simulink library "cooperative"  (Simulink 7.4)
settings: Solver=ode45  SolverMode=SingleTasking  StartTime=0.0  StopTime=10.0  RelTol=1e-3
undefined symbols (not defined in the file): ATRFunctions, g_AssignmentAlgorithm, g_CommandTurnRadius, g_CoordinationDelayDen, g_DefaultWaypointAltitude, g_EntityTypes, g_MaxNumberTargets, g_MaxNumberVehicles, g_MaxReassignmentDeltaTime, g_ObjectMessageIDs, g_OptionSaveDataAVDS, g_SampleTime, g_SensorRollLimitDeg, g_TargetStates, g_Tasks, g_TruthMemory, g_TypeAssignment, g_VehicleInputFiles, g_VehicleMemory, g_VehicleTypes, g_WaypointDefinitions, g_WaypointTypes
libraries: cooperative x23
(part 1 of 3)
settings Model: Creator=RAS  LastModifiedBy=z3311692  ExtModeAutoUpdateStatusClock=off

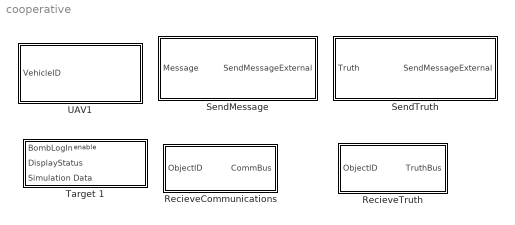
== system cooperative ==
  RecieveCommunications : Subsystem
  RecieveTruth : Subsystem
  SendMessage : Subsystem  mask{ReuseMatrix=growing, MessageTypeStr=ATRSingle}
      mask prompts: ReuseMatrix "Growing or Static memory matrix?"; MessageTypeStr "Select Message Type:"
      mask init:
      | global g_CommunicationMemory;
      | MessageIDIndex = FindMessageIndex(g_CommunicationMemory,MessageTypeStr);
      | MessageType = g_CommunicationMemory.Messages{MessageIDIndex}.ID;
      mask StyleString: popup(growing|static),popup(ETACostToSearch|PositionID|WaypointIndex|TriggerReplan|ATRSingle|ATRTime|TargetStatus|TargetAttacked|ChangedStatus|SendPositionsFlag|TaskBenefits|AuctionData)
  "SendTruth " : Subsystem  mask{ReuseMatrix=static, MessageTypeStr=VehicleState}
      mask prompts: ReuseMatrix "Growing or Static Memory Matrix?"; MessageTypeStr "Select Message Type:"
      mask init:
      | global g_TruthMemory
      | CommunicationsMemory = g_TruthMemory;
      | MessageIDIndex = FindMessageIndex(CommunicationsMemory ,MessageTypeStr);
      | MessageType = CommunicationsMemory.Messages{MessageIDIndex}.ID;
      mask StyleString: popup(growing|static),popup(VehicleState|VehicleIsDead|ChangeVehicleStatus|WeaponsRelease|TargetStatus|TargetState|VehicleStateSaveData|TrackList|ChangeAssignmentFlagSelf)
  Target 1 : Subsystem  AncestorBlock=cooperative/Target 1  TreatAsAtomicUnit=on
  UAV1 : Subsystem  Priority=2

== system cooperative/RecieveCommunications ==
  note: Communications Bus Simulation
      |
      | PURPOSE: Simulate communication subsystem.
      |
      | IMPLEMENTATION:
      | Vehicle-to-vehicle signals are isolated from the CommBus on CommBusSim.  In the case
      | of delayed communications, this is currently implimented with STL deques in the strigger files.
      | Strigger is essentially a trigger taking an arbitrary vector input that can be armed with a scalar
      | delay value...careful with those "enabled" blocks.
      |
      | See m-files:  GetVehicleCommDelay.m and InitializeGlobals.m for the OptionEnableCommDelay.
      |
      | NOTE:  YMMV.
  ObjectID : Inport
  Bus Creator1 : BusCreator  Inputs=24
  S-Function : S-Function  FunctionName=CommunicationsDLL  Parameters='g_CommunicationMemory'  EnableBusSupport=off
  CommBus : Outport
  wires:
  S-Function/24 -> Bus Creator1/24  "AuctionData"
  S-Function/23 -> Bus Creator1/23  "TimeAuctionData"
  S-Function/22 -> Bus Creator1/22  "TaskBenefits"
  S-Function/21 -> Bus Creator1/21  "TimeTaskBenefits"
  S-Function/20 -> Bus Creator1/20  "PositionsFlag"
  S-Function/19 -> Bus Creator1/19  "TimePositionsFlag"
  S-Function/18 -> Bus Creator1/18  "ChangedStatus"
  S-Function/17 -> Bus Creator1/17  "TimeChangedStatus"
  S-Function/16 -> Bus Creator1/16  "TargetAttacked"
  S-Function/15 -> Bus Creator1/15  "TimeTargetAttacked"
  S-Function/14 -> Bus Creator1/14  "TargetStatus"
  S-Function/13 -> Bus Creator1/13  "TimeTargetStatus"
  S-Function/12 -> Bus Creator1/12  "ATRTime"
  S-Function/11 -> Bus Creator1/11  "TimeATRTime"
  S-Function/10 -> Bus Creator1/10  "ATRSingle"
  S-Function/9 -> Bus Creator1/9  "TimeATRSingle"
  S-Function/8 -> Bus Creator1/8  "TriggerReplan"
  S-Function/7 -> Bus Creator1/7  "TimeTriggerReplan"
  S-Function/6 -> Bus Creator1/6  "WaypointIndex"
  S-Function/5 -> Bus Creator1/5  "TimeWaypointIndex"
  S-Function/4 -> Bus Creator1/4  "PositionID"
  S-Function/3 -> Bus Creator1/3  "TimePositionID"
  S-Function/2 -> Bus Creator1/2  "ETACostToSearch"
  S-Function/1 -> Bus Creator1/1  "TimeETACostToSearch"
  ObjectID/1 -> S-Function/1
  Bus Creator1/1 -> CommBus/1  "ExternalComm"

== system cooperative/RecieveTruth ==
  note: Communications Bus Simulation
      |
      | PURPOSE: Simulate communication subsystem.
      |
      | IMPLEMENTATION:
      | Vehicle-to-vehicle signals are isolated from the CommBus on CommBusSim.  In the case
      | of delayed communications, this is currently implimented with STL deques in the strigger files.
      | Strigger is essentially a trigger taking an arbitrary vector input that can be armed with a scalar
      | delay value...careful with those "enabled" blocks.
      |
      | See m-files:  GetVehicleCommDelay.m and InitializeGlobals.m for the OptionEnableCommDelay.
      |
      | NOTE:  YMMV.
  ObjectID : Inport
  Bus Creator1 : BusCreator  Inputs=18
  S-Function : S-Function  FunctionName=CommunicationsDLL  Parameters='g_TruthMemory'  EnableBusSupport=off
  TruthBus : Outport
  wires:
  S-Function/18 -> Bus Creator1/18  "ChangeAssignmentFlagSelf"
  S-Function/17 -> Bus Creator1/17  "TimeChangeAssignmentFlagSelf"
  S-Function/16 -> Bus Creator1/16  "TrackList"
  S-Function/15 -> Bus Creator1/15  "TimeTrackList"
  S-Function/14 -> Bus Creator1/14  "VehicleStateSaveData"
  S-Function/13 -> Bus Creator1/13  "TimeVehicleStateSaveData"
  S-Function/12 -> Bus Creator1/12  "TargetState"
  S-Function/11 -> Bus Creator1/11  "TimeTargetState"
  S-Function/2 -> Bus Creator1/2  "VehicleStates"
  S-Function/1 -> Bus Creator1/1  "TimeVehicleStates"
  S-Function/3 -> Bus Creator1/3  "TimeVehicleIsDead"
  S-Function/4 -> Bus Creator1/4  "VehicleIsDead"
  S-Function/5 -> Bus Creator1/5  "TimeVehicleKilled"
  S-Function/6 -> Bus Creator1/6  "VehicleKilled"
  S-Function/7 -> Bus Creator1/7  "TimeWeaponRelease"
  S-Function/8 -> Bus Creator1/8  "WeaponRelease"
  S-Function/9 -> Bus Creator1/9  "TimeTargetStatus"
  S-Function/10 -> Bus Creator1/10  "TargetStatus"
  ObjectID/1 -> S-Function/1
  Bus Creator1/1 -> TruthBus/1  "ExternalTruth"

== system cooperative/SendMessage ==
  Message : Inport
  Check for Changed Targets : RelationalOperator  Operator=~=  InputSameDT=on
  CreateLastTriggerTime : DataStoreMemory  DataStoreName=LastTriggerTime
  ReadLastTriggerTime : DataStoreRead  DataStoreName=LastTriggerTime  SampleTime=g_SampleTime
  Selector : Selector  IndexOptions=Index vector (dialog)  Indices=2  OutputSizes=1
  SendMessage : Subsystem  TreatAsAtomicUnit=on
  SendMessageExternal : Outport
  wires:
  Message/1 -> Selector/1, SendMessage/2(Message)
  Check for Changed Targets/1 -> SendMessage/Enable
  ReadLastTriggerTime/1 -> Check for Changed Targets/1
  Selector/1 -> Check for Changed Targets/2, SendMessage/1(ReplanTime)
  SendMessage/1(SendMessageExternal) -> SendMessageExternal/1  "SendMessage"

== system cooperative/SendTruth  ==
  Truth : Inport
  Check for Changed Targets : RelationalOperator  Operator=~=  InputSameDT=on
  CreateLastTriggerTime : DataStoreMemory  DataStoreName=LastTriggerTime
  ReadLastTriggerTime : DataStoreRead  DataStoreName=LastTriggerTime  SampleTime=g_SampleTime
  Selector : Selector  IndexOptions=Index vector (dialog)  Indices=2  OutputSizes=1
  SendMessage : Subsystem  TreatAsAtomicUnit=on
  SendMessageExternal : Outport
  wires:
  Selector/1 -> Check for Changed Targets/2, SendMessage/1(ReplanTime)
  ReadLastTriggerTime/1 -> Check for Changed Targets/1
  Check for Changed Targets/1 -> SendMessage/Enable
  Truth/1 -> Selector/1, SendMessage/2(Message)
  SendMessage/1(SendMessageExternal) -> SendMessageExternal/1  "SendMessage"

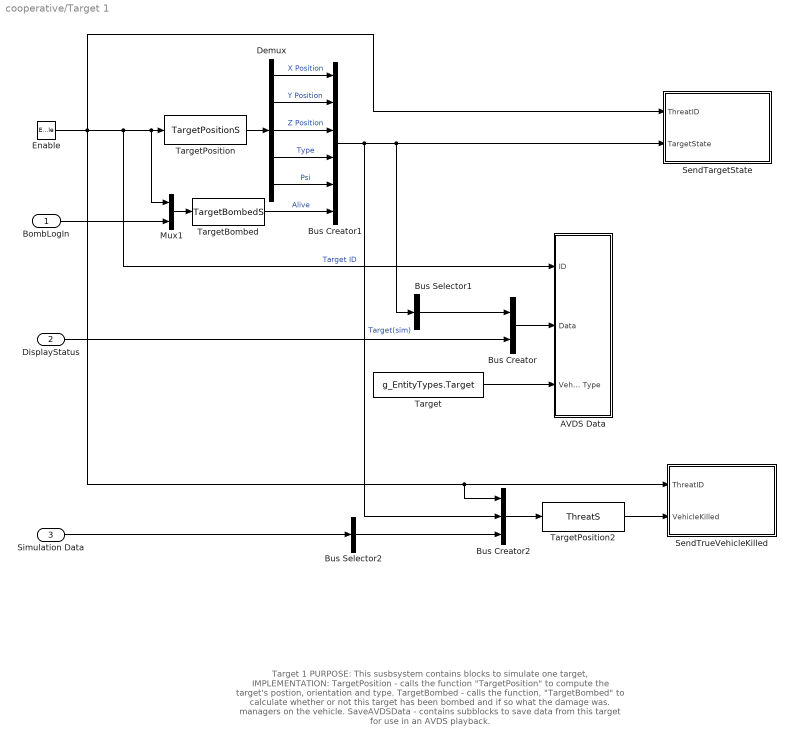
== system cooperative/Target 1 ==
  note: Target 1
      |
      | PURPOSE: This susbsystem contains blocks to simulate one target,
      |
      | IMPLEMENTATION:
      | TargetPosition - calls the function "TargetPosition" to compute the target's postion,
      |      orientation and type.
      | TargetBombed - calls the function, "TargetBombed" to calculate whether or not this
      |      target has been bombed and if so what the damage was.
      |      managers on the vehicle.
      | SaveAVDSData - contains subblocks to save data from this target for use
      |     in an AVDS playback.
  BombLogIn : Inport  SampleTime=g_SampleTime
  DisplayStatus : Inport  Port=2  SampleTime=g_SampleTime
  Simulation Data : Inport  Port=3  SampleTime=g_SampleTime
  Enable : EnablePort  StatesWhenEnabling=reset  ShowOutputPort=on
  AVDS Data : Subsystem
  Bus Creator : BusCreator  Inputs=2
  Bus Creator1 : BusCreator  Inputs=6
  Bus Creator2 : BusCreator  Inputs=3
  Bus Selector1 : BusSelector  OutputSignals=X Position,Y Position,Z Position,Type,Psi  OutputAsBus=on
  Bus Selector2 : BusSelector  OutputSignals=VehicleStates  OutputAsBus=on
  Demux : Demux  Outputs=5
  Mux1 : Mux  Inputs=2
  SendTargetState : Subsystem
  SendTrueVehicleKilled : Subsystem
  Target : Constant  Value=g_EntityTypes.Target
  TargetBombed : S-Function  FunctionName=TargetBombedS  EnableBusSupport=off
  TargetPosition : S-Function  FunctionName=TargetPositionS  EnableBusSupport=off
  TargetPosition2 : S-Function  FunctionName=ThreatS  Parameters=g_MaxNumberVehicles  EnableBusSupport=off
  wires:
  Enable/1 -> AVDS Data/1(ID), Mux1/1, TargetPosition/1, Bus Creator2/1, SendTrueVehicleKilled/1(ThreatID), SendTargetState/1(ThreatID)  "Target ID"
  TargetPosition/1 -> Demux/1
  Target/1 -> AVDS Data/3(Vehicle Type)
  Bus Selector1/1 -> Bus Creator/1
  Demux/1 -> Bus Creator1/1  "X Position"
  Demux/2 -> Bus Creator1/2  "Y Position"
  Demux/3 -> Bus Creator1/3  "Z Position"
  Bus Creator1/1 -> Bus Selector1/1, SendTargetState/2(TargetState), Bus Creator2/2  "Target(sim)"
  Demux/5 -> Bus Creator1/5  "Psi"
  BombLogIn/1 -> Mux1/2
  Demux/4 -> Bus Creator1/4  "Type"
  TargetBombed/1 -> Bus Creator1/6  "Alive"
  Mux1/1 -> TargetBombed/1
  Bus Creator/1 -> AVDS Data/2(Data)
  DisplayStatus/1 -> Bus Creator/2
  TargetPosition2/1 -> SendTrueVehicleKilled/2(VehicleKilled)
  Bus Creator2/1 -> TargetPosition2/1
  Bus Selector2/1 -> Bus Creator2/3
  Simulation Data/1 -> Bus Selector2/1

== system cooperative/UAV1 ==
  note: UAV1
      |
      | PURPOSE: This susbsystem contains blocks to simulate one vehicle,
      |
      | IMPLEMENTATION:
      | Aircraft Dynamics - contains subblocks to implement the vehicle's dynamics
      |      simulation.
      | Embedded Flight Software - contains subblocks to implement the software
      |      managers on the vehicle.
      | SaveAVDSData - contains subblocks to save data from this ehicle for use
      |     in an AVDS playback.
  VehicleID : Inport  SampleTime=g_SampleTime
  Aircraft Dynamics : Subsystem  TreatAsAtomicUnit=on
  Bus Creator : BusCreator  Inputs=1
  Bus Creator1 : BusCreator
  Bus Creator4 : BusCreator  Inputs=1
  Digital Clock : DigitalClock  SampleTime=g_SampleTime
  EmbeddedFlightSoftware : Subsystem
  ReceiveMessages : Subsystem
  ReceiveTruth : Subsystem
  SaveAVDSData : Subsystem
  SendMessages : Subsystem
  SendTruth : Subsystem
  wires:
  ReceiveMessages/1(CommBusSim Out) -> SendMessages/3(CommBus), EmbeddedFlightSoftware/2(ComBusIn)
  Digital Clock/1 -> Bus Creator1/2  "Time"
  EmbeddedFlightSoftware/2(ComBusOut) -> Bus Creator1/4
  EmbeddedFlightSoftware/1(SimBusOut) -> Bus Creator/1
  VehicleID/1 -> ReceiveMessages/1(VehicleID), SaveAVDSData/1(ID), EmbeddedFlightSoftware/5(Enable), ReceiveTruth/1(Vehicle ID), Bus Creator1/1, SendMessages/1(VehicleID), SendTruth/1(VehicleID), Aircraft Dynamics/Enable  "VehicleID"
  Bus Creator/1 -> SaveAVDSData/3(SimBusLocalln), EmbeddedFlightSoftware/3(SimBusLocalIn), SendTruth/3(SimmBusLocal)  "SimBusLocal"
  Bus Creator1/1 -> SaveAVDSData/2(ComBusLocalln), EmbeddedFlightSoftware/4(ComBusLocalIn), Aircraft Dynamics/2(ComBusLocalIn), SendMessages/2(CommBusLocal), SendTruth/2(CommBusLocal)  "ComBusLocal"
  Aircraft Dynamics/1(ComBusOut) -> Bus Creator1/3
  Bus Creator4/1 -> Aircraft Dynamics/1(SimBusIn), EmbeddedFlightSoftware/1(SimBusIn)
  ReceiveTruth/1(TruthBusOut) -> Bus Creator4/1

== system cooperative/SendMessage/SendMessage ==
  ReplanTime : Inport
  Message : Inport  Port=2
  Enable : EnablePort
  Constant : Constant  Value=g_TruthMemory.Transport.MatlabMatrix
  Constant1 : Constant  Value=g_TruthMemory.Transport.TransportType
  Relational Operator : RelationalOperator  Operator===  InputSameDT=on
  SaveLastTriggerTime : DataStoreWrite  DataStoreName=LastTriggerTime  SampleTime=g_SampleTime
  SendMessageMatlab : Subsystem  TreatAsAtomicUnit=on
  SendMessageExternal : Outport
  wires:
  Constant1/1 -> Relational Operator/2
  Constant/1 -> Relational Operator/1
  Relational Operator/1 -> SendMessageMatlab/Enable
  Message/1 -> SendMessageExternal/1, SendMessageMatlab/1(Message)
  ReplanTime/1 -> SaveLastTriggerTime/1

== system cooperative/SendTruth /SendMessage ==
  ReplanTime : Inport
  Message : Inport  Port=2
  Enable : EnablePort
  Constant : Constant  Value=g_TruthMemory.Transport.MatlabMatrix
  Constant1 : Constant  Value=g_TruthMemory.Transport.TransportType
  Relational Operator : RelationalOperator  Operator===  InputSameDT=on
  SaveLastTriggerTime : DataStoreWrite  DataStoreName=LastTriggerTime  SampleTime=g_SampleTime
  SendMessageMatlab : Subsystem  TreatAsAtomicUnit=on
  SendMessageExternal : Outport
  wires:
  ReplanTime/1 -> SaveLastTriggerTime/1
  Message/1 -> SendMessageMatlab/1(Message), SendMessageExternal/1
  Relational Operator/1 -> SendMessageMatlab/Enable
  Constant/1 -> Relational Operator/1
  Constant1/1 -> Relational Operator/2

== system cooperative/Target 1/AVDS Data ==
  note: AVDS Data
      |
      | PURPOSE: Save target state information to a text file that is suitable
      |      for playback in AVDS.
      |
      | IMPLEMENTATION:
      | - Save Target Data for AVDS - calls the function "AVDSData2WorkSpace"
      |      to save the data.
      | - NotAtZero - data saving is enabled when the simulation time is greater
      |      than 0.0 to prevent unitialized data from being written to the file.
      | - EnableDataSaving - reads the global array "OptionSaveDataAVDS" to
      |      enable/disable data saving.
  ID : Inport  SampleTime=g_SampleTime
  Data : Inport  Port=2  SampleTime=g_SampleTime
  Vehicle Type : Inport  Port=3  SampleTime=g_SampleTime
  Digital Clock : DigitalClock  SampleTime=g_SampleTime
  EnableDataSaving : Constant  Value=g_OptionSaveDataAVDS
  Logical Operator : Logic
  NotAtZero : Fcn  Expr=u(1) > 0
  SaveTarget  Data for AVDS : Subsystem  TreatAsAtomicUnit=on
  wires:
  ID/1 -> SaveTarget  Data for AVDS/2(ID)
  Data/1 -> SaveTarget  Data for AVDS/3(Data)
  Digital Clock/1 -> NotAtZero/1, SaveTarget  Data for AVDS/1(Time)
  Vehicle Type/1 -> SaveTarget  Data for AVDS/4(Vehicle Type)
  NotAtZero/1 -> Logical Operator/2
  Logical Operator/1 -> SaveTarget  Data for AVDS/Enable
  EnableDataSaving/1 -> Logical Operator/1

== system cooperative/Target 1/SendTargetState ==
  ThreatID : Inport
  TargetState : Inport  Port=2
  Constant : Constant  Value=0
  CreateTargetState : DataStoreMemory  DataStoreName=TargetState  InitialValue=zeros(6,1)
  Enabled Subsystem : Subsystem  TreatAsAtomicUnit=on
  Logical Operator : Logic  Operator=OR
  Mux2 : Mux  Inputs=3
  ReadTargetState : DataStoreRead  DataStoreName=TargetState  SampleTime=g_SampleTime
  Relational Operator : RelationalOperator  Operator=~=  InputSameDT=on
  Relational Operator1 : RelationalOperator  Operator===  InputSameDT=on
  "SendTruth " : cooperative/SendTruth   ReuseMatrix=static  MessageTypeStr=TargetState
  Terminator : Terminator
  Unit Delay : UnitDelay  SampleTime=g_SampleTime
  wires:
  Relational Operator/1 -> Logical Operator/1
  Enabled Subsystem/1(TimeStamp) -> Unit Delay/1, Mux2/2
  ReadTargetState/1 -> Relational Operator/1
  TargetState/1 -> Enabled Subsystem/1(TargetState), Relational Operator/2, Mux2/3
  ThreatID/1 -> Mux2/1
  Mux2/1 -> "SendTruth "/1
  Logical Operator/1 -> Enabled Subsystem/Enable
  Relational Operator1/1 -> Logical Operator/2
  Constant/1 -> Relational Operator1/1
  Unit Delay/1 -> Relational Operator1/2
  "SendTruth "/1 -> Terminator/1

== system cooperative/Target 1/SendTrueVehicleKilled ==
  ThreatID : Inport
  VehicleKilled : Inport  Port=2
  CreateVehicleKilled : DataStoreMemory  DataStoreName=VehicleKilled  InitialValue=zeros(g_MaxNumberVehicles,1)
  Enabled Subsystem : Subsystem  TreatAsAtomicUnit=on
  Mux2 : Mux
  ReadVehicleKilled : DataStoreRead  DataStoreName=VehicleKilled  SampleTime=g_SampleTime
  Recipients : Constant  Value=g_ObjectMessageIDs.AllVehiclesTypeShifted + 1
  Relational Operator : RelationalOperator  Operator=~=  InputSameDT=on
  "SendTruth " : cooperative/SendTruth   ReuseMatrix=growing  MessageTypeStr=ChangeVehicleStatus
  Terminator : Terminator
  wires:
  Mux2/1 -> "SendTruth "/1
  ThreatID/1 -> Mux2/1
  VehicleKilled/1 -> Mux2/3, Relational Operator/2, Enabled Subsystem/1(VehicleKilled)
  ReadVehicleKilled/1 -> Relational Operator/1
  Enabled Subsystem/1(TimeStamp) -> Mux2/2
  Relational Operator/1 -> Enabled Subsystem/Enable
  Recipients/1 -> Mux2/4
  "SendTruth "/1 -> Terminator/1

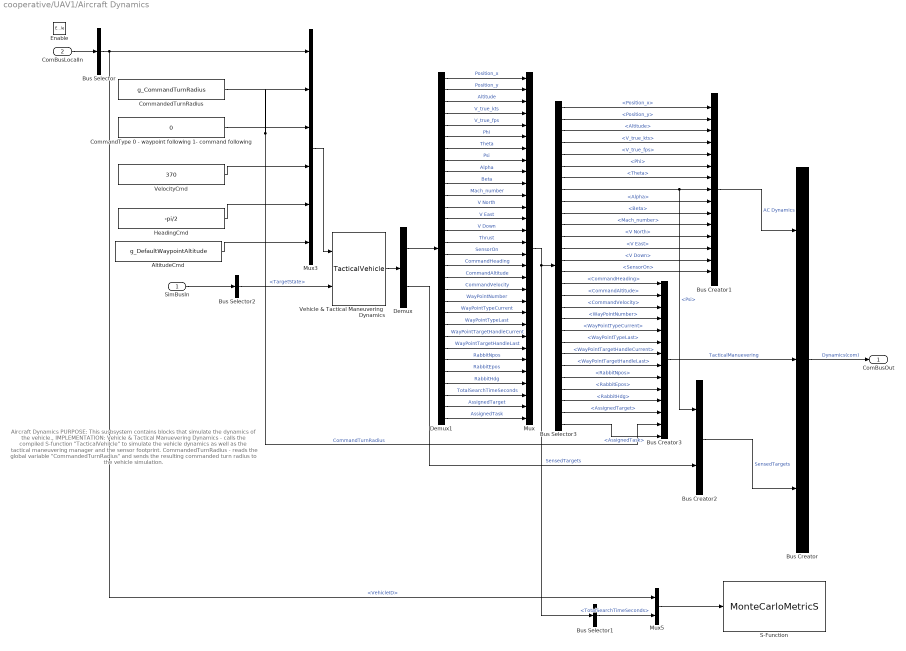
== system cooperative/UAV1/Aircraft Dynamics ==
  note: Aircraft Dynamics
      |
      | PURPOSE: This susbsystem contains blocks that simulate the dynamics of the vehicle.,
      |
      | IMPLEMENTATION:
      | Vehicle & Tactical Manuevering Dynamics - calls the compiled S-function "TacticalVehilcle"
      |      to simulate the vehicle dynamics as well as the tactical maneuvering manager and the
      |      sensor footprint.
      | CommandedTurnRadius - reads the global variable "CommandedTurnRadius" and sends
      |      the resulting commanded turn radius to the vehicle simulation.
  SimBusIn : Inport  SampleTime=g_SampleTime
  ComBusLocalIn : Inport  Port=2  SampleTime=g_SampleTime
  Enable : EnablePort
  AltitudeCmd : Constant  Value=g_DefaultWaypointAltitude
  Bus Creator : BusCreator  Inputs=3
  Bus Creator1 : BusCreator  Inputs=15
  Bus Creator2 : BusCreator  Inputs=2
  Bus Creator3 : BusCreator  Inputs=14
  Bus Selector : BusSelector  OutputSignals=VehicleID
  Bus Selector1 : BusSelector  OutputSignals=TotalSearchTimeSeconds
  Bus Selector2 : BusSelector  OutputSignals=ExternalTruth.TargetState
  Bus Selector3 : BusSelector  OutputSignals=Position_x,Position_y,Altitude,V_true_kts,V_true_fps,Phi,Theta,Psi,Alpha,Beta,Mach_number,V North,V East,V Down,SensorOn,CommandHeading,CommandAltitude,CommandVelocity,WayPointNumber,WayPointTypeCurrent,WayPointTypeLast,WayPointTargetHandleCurrent,WayPointTargetHandleLast,RabbitNpos,RabbitEpos,RabbitHdg,AssignedTarget,AssignedTask
  CommandType 0 - waypoint following 1- command following : Constant  Value=0
  CommandedTurnRadius : Constant  Value=g_CommandTurnRadius
  Demux : Demux  Outputs=[30 g_MaxNumberTargets]
  Demux1 : Demux  Outputs=30
  HeadingCmd : Constant  Value=-pi/2
  Mux : Mux  Inputs=30
  Mux3 : Mux  Inputs=6
  Mux5 : Mux  Inputs=2
  S-Function : S-Function  FunctionName=MonteCarloMetricS  Parameters='TotalSearchTimeSeconds'  EnableBusSupport=off
  Vehicle & Tactical Maneuvering  Dynamics : S-Function  FunctionName=TacticalVehicle  Parameters=0,g_MaxNumberTargets,g_SensorRollLimitDeg,g_WaypointDefinitions.NumberEntries,g_VehicleInputFiles  EnableBusSupport=off
  VelocityCmd : Constant  Value=370
  ComBusOut : Outport
  wires:
  Bus Selector1/1 -> Mux5/2  "<TotalSearchTimeSeconds>"
  Mux5/1 -> S-Function/1
  Demux1/25 -> Mux/25  "RabbitNpos"
  Demux1/30 -> Mux/30  "AssignedTask"
  ComBusLocalIn/1 -> Bus Selector/1
  SimBusIn/1 -> Bus Selector2/1
  Bus Creator3/1 -> Bus Creator/2  "TacticalManuevering"
  Mux/1 -> Bus Selector1/1, Bus Selector3/1
  Bus Selector3/15 -> Bus Creator1/15  "<SensorOn>"
  Bus Creator1/1 -> Bus Creator/1  "AC Dynamics"
  Bus Selector3/14 -> Bus Creator1/14  "<V Down>"
  Bus Selector3/13 -> Bus Creator1/13  "<V East>"
  Bus Selector3/12 -> Bus Creator1/12  "<V North>"
  Bus Selector3/11 -> Bus Creator1/11  "<Mach_number>"
  Bus Selector3/10 -> Bus Creator1/10  "<Beta>"
  Bus Selector3/9 -> Bus Creator1/9  "<Alpha>"
  Bus Selector3/8 -> Bus Creator1/8, Bus Creator2/1  "<Psi>"
  Bus Selector3/7 -> Bus Creator1/7  "<Theta>"
  Bus Selector3/6 -> Bus Creator1/6  "<Phi>"
  Bus Selector3/5 -> Bus Creator1/5  "<V_true_fps>"
  Bus Selector3/4 -> Bus Creator1/4  "<V_true_kts>"
  Bus Selector3/3 -> Bus Creator1/3  "<Altitude>"
  Bus Selector3/2 -> Bus Creator1/2  "<Position_y>"
  Bus Selector3/1 -> Bus Creator1/1  "<Position_x>"
  Demux1/29 -> Mux/29  "AssignedTarget"
  Demux1/27 -> Mux/27  "RabbitHdg"
  Demux1/26 -> Mux/26  "RabbitEpos"
  Demux1/22 -> Mux/22  "WayPointTypeLast"
  Demux1/21 -> Mux/21  "WayPointTypeCurrent"
  Demux1/20 -> Mux/20  "WayPointNumber"
  Demux1/19 -> Mux/19  "CommandVelocity"
  Demux1/18 -> Mux/18  "CommandAltitude"
  Demux1/17 -> Mux/17  "CommandHeading"
  Demux1/16 -> Mux/16  "SensorOn"
  Demux1/15 -> Mux/15  "Thrust"
  Demux1/14 -> Mux/14  "V Down"
  Demux1/13 -> Mux/13  "V East"
  Demux1/12 -> Mux/12  "V North"
  Demux1/11 -> Mux/11  "Mach_number"
  Demux1/10 -> Mux/10  "Beta"
  Demux1/9 -> Mux/9  "Alpha"
  Demux1/8 -> Mux/8  "Psi"
  Demux1/7 -> Mux/7  "Theta"
  Demux1/6 -> Mux/6  "Phi"
  Demux1/5 -> Mux/5  "V_true_fps"
  Demux1/4 -> Mux/4  "V_true_kts"
  Demux1/2 -> Mux/2  "Position_y"
  Demux1/1 -> Mux/1  "Position_x"
  Demux1/3 -> Mux/3  "Altitude"
  Demux/2 -> Bus Creator2/2  "SensedTargets"
  Demux/1 -> Demux1/1
  Bus Creator2/1 -> Bus Creator/3  "SensedTargets"
  Bus Creator/1 -> ComBusOut/1  "Dynamics(com)"
  CommandedTurnRadius/1 -> Bus Creator3/13, Mux3/2  "CommandTurnRadius"
  Bus Selector/1 -> Mux5/1, Mux3/1  "<VehicleID>"
  Vehicle & Tactical Maneuvering  Dynamics/1 -> Demux/1
  Bus Selector2/1 -> Vehicle & Tactical Maneuvering  Dynamics/2  "<TargetState>"
  Mux3/1 -> Vehicle & Tactical Maneuvering  Dynamics/1
  Demux1/23 -> Mux/23  "WayPointTargetHandleCurrent"
  Demux1/24 -> Mux/24  "WayPointTargetHandleLast"
  Demux1/28 -> Mux/28  "TotalSearchTimeSeconds"
  Bus Selector3/16 -> Bus Creator3/1  "<CommandHeading>"
  Bus Selector3/17 -> Bus Creator3/2  "<CommandAltitude>"
  Bus Selector3/18 -> Bus Creator3/3  "<CommandVelocity>"
  Bus Selector3/19 -> Bus Creator3/4  "<WayPointNumber>"
  Bus Selector3/20 -> Bus Creator3/5  "<WayPointTypeCurrent>"
  Bus Selector3/21 -> Bus Creator3/6  "<WayPointTypeLast>"
  Bus Selector3/22 -> Bus Creator3/7  "<WayPointTargetHandleCurrent>"
  Bus Selector3/23 -> Bus Creator3/8  "<WayPointTargetHandleLast>"
  Bus Selector3/24 -> Bus Creator3/9  "<RabbitNpos>"
  Bus Selector3/25 -> Bus Creator3/10  "<RabbitEpos>"
  Bus Selector3/26 -> Bus Creator3/11  "<RabbitHdg>"
  Bus Selector3/27 -> Bus Creator3/12  "<AssignedTarget>"
  Bus Selector3/28 -> Bus Creator3/14  "<AssignedTask>"
  CommandType 0 - waypoint following 1- command following/1 -> Mux3/3
  VelocityCmd/1 -> Mux3/4
  HeadingCmd/1 -> Mux3/5
  AltitudeCmd/1 -> Mux3/6

== system cooperative/UAV1/EmbeddedFlightSoftware ==
  note: EmbeddedFlightSoftware
      |
      | PURPOSE: This susbsystem contains subsystems to implement the software
      |      managers on the vehicle,
      |
      | IMPLEMENTATION:
      | - Sensor Manager -  This manager is used to perform all of the functions
      |      necessary to monitor the sensors and process sensed data.
      | - TargetManager - Tracks and updates the status of all kown targets.
      | - WeaponsManager - Selects a weapon and then simulates its deployment.
      | - CooperationManager - This manager is used to facilitate cooperation
      |      between the vehicles. At this time the only function implemented is the
      |      Assginment manager.
      | - RouteManager - This manager is used to plan and select the route
      |      for the vehicle to fly. Part of the functionality is calculation of the lowest
      |      cost route to all known targets, based on each target's state.
  SimBusIn : Inport  SampleTime=g_SampleTime
  ComBusIn : Inport  Port=2  SampleTime=g_SampleTime
  SimBusLocalIn : Inport  Port=3  SampleTime=g_SampleTime
  ComBusLocalIn : Inport  Port=4  SampleTime=g_SampleTime
  Enable : Inport  Port=5  SampleTime=g_SampleTime
  Bus Creator : BusCreator  Inputs=3
  Bus Creator1 : BusCreator  Inputs=5
  CooperationManager : Subsystem
  RouteManager : Subsystem
  SensorManager : Subsystem
  TargetManager : Subsystem
  TimeLastReplan1 : DataStoreMemory  DataStoreName=TimeLastReplan
  WeaponsManager : Subsystem  TreatAsAtomicUnit=on
  SimBusOut : Outport
  ComBusOut : Outport  Port=2
  wires:
  Enable/1 -> RouteManager/5(Enable), CooperationManager/4(Enable), WeaponsManager/Enable, SensorManager/4(Enable), TargetManager/4(Enable)
  RouteManager/2(ComBusOut) -> Bus Creator1/5
  CooperationManager/1(ComBusOut) -> Bus Creator1/4
  WeaponsManager/2(ComBusOut) -> Bus Creator1/3
  TargetManager/1(ComBusOut) -> Bus Creator1/2
  SensorManager/1(ComBusOut) -> Bus Creator1/1
  RouteManager/1(SimBusOut) -> Bus Creator/3
  WeaponsManager/1(SimBusOut) -> Bus Creator/1
  Bus Creator/1 -> SimBusOut/1  "EFS(sim)"
  Bus Creator1/1 -> ComBusOut/1  "EFS(com)"
  SimBusIn/1 -> TargetManager/1(SimBusIn), SensorManager/1(SimBusIn), CooperationManager/1(SimBusIn), RouteManager/1(SimBusIn)
  ComBusIn/1 -> TargetManager/2(ComBusIn), SensorManager/2(ComBusIn), CooperationManager/2(ComBusIn), RouteManager/2(ComBusIn)
  SimBusLocalIn/1 -> RouteManager/3(SimBusLocalIn)
  ComBusLocalIn/1 -> WeaponsManager/1(ComBusLocalIn), TargetManager/3(ComBusLocalIn), SensorManager/3(ComBusLocalIn), CooperationManager/3(ComBusLocalIn), RouteManager/4(ComBusLocalIn)
  CooperationManager/2(SimBusOut) -> Bus Creator/2

== system cooperative/UAV1/ReceiveMessages ==
  VehicleID : Inport
  RecieveCommunications : cooperative/RecieveCommunications
      settings: RTWFcnNameOpts=Auto  RTWFileNameOpts=Auto
  Sum : Sum  Inputs=|++  SaturateOnIntegerOverflow=on  InputSameDT=on  OutDataTypeStr=Inherit: Same as first input
  VehicleOffset : Constant  Value=g_ObjectMessageIDs.VehicleIDOffset
  CommBusSim Out : Outport
  wires:
  RecieveCommunications/1 -> CommBusSim Out/1
  VehicleID/1 -> Sum/1
  VehicleOffset/1 -> Sum/2
  Sum/1 -> RecieveCommunications/1

== system cooperative/UAV1/ReceiveTruth ==
  Vehicle ID : Inport
  ImplementNewAssignment : Subsystem
  RecieveTruth : cooperative/RecieveTruth
      settings: RTWFcnNameOpts=Auto  RTWFileNameOpts=Auto
  Sum : Sum  Inputs=|+|+|  SaturateOnIntegerOverflow=on  InputSameDT=on  OutDataTypeStr=Inherit: Same as first input
  VehicleOffset : Constant  Value=g_ObjectMessageIDs.VehicleIDOffset
  TruthBusOut : Outport
  wires:
  RecieveTruth/1 -> TruthBusOut/1, ImplementNewAssignment/2(TruthBus)
  Vehicle ID/1 -> ImplementNewAssignment/1(VehicleID), Sum/2
  Sum/1 -> RecieveTruth/1
  VehicleOffset/1 -> Sum/1

== system cooperative/UAV1/SaveAVDSData ==
  note: AVDS Data
      |
      | PURPOSE: Save vehicle state information to a
      | text file that is suitable for playback in AVDS.
      |
      | IMPLEMENTATION:
      | - SaveVehicleData for AVDS - calls the function "AVDSData2WorkSpace"
      |      to save the data.
      | - NotAtZero - data saving is enabled when the simulation time is greater
      |      than 0.0 to prevent unitialized data from being written to the file.
      | -EnableDataSaving - reads the global array "OptionSaveDataAVDS" to
      |      enables/disables saving data forAVDS.
  ID : Inport  SampleTime=g_SampleTime
  ComBusLocalln : Inport  Port=2  SampleTime=g_SampleTime
  SimBusLocalln : Inport  Port=3  SampleTime=g_SampleTime
  Aircraft : Constant  Value=g_EntityTypes.Aircraft
  Bus Selector2 : BusSelector  OutputSignals=Dynamics(com).AC Dynamics.Position_x,Dynamics(com).AC Dynamics.Position_y,Dynamics(com).AC Dynamics.Altitude,Dynamics(com).AC Dynamics.Phi,Dynamics(com).AC Dynamics.Theta,Dynamics(com).AC Dynamics.Psi,Dynamics(com).AC Dynamics.Alpha,Dynamics(com).AC Dynamics.Beta,Dynamics(com).AC Dynamics.V_true_fps,Dynamics(com).AC Dynamics.Mach_number,Dynamics(com).TacticalManuevering.AssignedTarget,Dynamics(com).TacticalManuevering.AssignedTask,Dynamics(com).TacticalManuevering.RabbitNpos,Dynamics(com).TacticalManuevering.RabbitEpos,Dynamics(com).TacticalManuevering.RabbitHdg,Dynamics(com).TacticalManuevering.CommandAltitude,Dynamics(com).AC Dynamics.SensorOn  OutputAsBus=on
  Bus Selector3 : BusSelector  OutputSignals=EFS(sim).RouteManager(sim).VehicleFinished.Vehicle FinishedNoDelay
  Digital Clock : DigitalClock  SampleTime=g_SampleTime
  "EnableDataSaving " : Constant  Value=g_OptionSaveDataAVDS
  Logical Operator : Logic  Inputs=3
  Mux4 : Mux  Inputs=2
  NotAtZero : Fcn  Expr=u(1) > g_SampleTime
  SaveVehicleData for AVDS : Subsystem  TreatAsAtomicUnit=on
  wires:
  NotAtZero/1 -> Logical Operator/3
  Aircraft/1 -> SaveVehicleData for AVDS/4(Vehicle Type)
  Digital Clock/1 -> SaveVehicleData for AVDS/1(Time), NotAtZero/1
  SimBusLocalln/1 -> Bus Selector3/1
  ComBusLocalln/1 -> Bus Selector2/1
  ID/1 -> SaveVehicleData for AVDS/2(ID), Logical Operator/2
  Logical Operator/1 -> SaveVehicleData for AVDS/Enable
  "EnableDataSaving "/1 -> Logical Operator/1
  Bus Selector2/1 -> Mux4/1
  Bus Selector3/1 -> Mux4/2  "<Vehicle FinishedNoDelay>"
  Mux4/1 -> SaveVehicleData for AVDS/3(Data)

== system cooperative/UAV1/SendMessages ==
  note: Messages must have elements starting with vehicleid,timestamp,...
  VehicleID : Inport
  CommBusLocal : Inport  Port=2
  CommBus : Inport  Port=3
  SendATRSingle : Subsystem
  SendATRTime : Subsystem
  SendAuctionData : Subsystem
  SendChangedStatus : Subsystem
  SendETAsCostsReturnToSearch : Subsystem
  SendPositionFlag : Subsystem
  SendPositionID : Subsystem
  SendTargetAttacked : Subsystem
  SendTargetStatus : Subsystem
  SendTaskBenefits : Subsystem
  SendTriggerReplan : Subsystem  Priority=1
  SendWaypointNumber : Subsystem
  wires:
  CommBus/1 -> SendPositionFlag/3(CommBus), SendPositionID/3(CommBus)
  CommBusLocal/1 -> SendATRTime/2(CommBusLocal), SendATRSingle/2(CommBusLocal), SendETAsCostsReturnToSearch/2(CommBusLocal), SendTriggerReplan/2(CommBusLocal), SendAuctionData/2(CommBusLocal), SendTaskBenefits/2(CommBusLocal), SendPositionFlag/2(CommBusLocal), SendPositionID/2(CommBusLocal), SendTargetStatus/2(CommBusLocal), SendTargetAttacked/2(CommBusLocal), SendChangedStatus/2(CommBusLocal), SendWaypointNumber/2(CommBusLocal)
  VehicleID/1 -> SendETAsCostsReturnToSearch/1(VehicleID), SendTriggerReplan/1(VehicleID), SendATRTime/1(VehicleID), SendAuctionData/1(VehicleID), SendTaskBenefits/1(VehicleID), SendPositionFlag/1(VehicleID), SendPositionID/1(VehicleID), SendTargetStatus/1(VehicleID), SendTargetAttacked/1(VehicleID), SendChangedStatus/1(VehicleID), SendWaypointNumber/1(VehicleID), SendATRSingle/1(VehicleID)

== system cooperative/UAV1/SendTruth ==
  note: Messages must have elements starting with vehicleid,timestamp,...
  VehicleID : Inport
  CommBusLocal : Inport  Port=2
  SimmBusLocal : Inport  Port=3
  SendNewAssignment : Subsystem
  SendTargetStatus : Subsystem
  SendTrackList : Subsystem
  SendTrueVehicleState : Subsystem
  SendVehicleIsDead : Subsystem
  SendWeaponsRelease : Subsystem
  VehicleStateSaveData : Subsystem
  wires:
  VehicleID/1 -> SendVehicleIsDead/1(VehicleID), SendWeaponsRelease/1(VehicleID), SendTargetStatus/1(VehicleID), VehicleStateSaveData/1(VehicleID), SendTrackList/1(VehicleID), SendTrueVehicleState/1(VehicleID), SendNewAssignment/1(VehicleID)
  CommBusLocal/1 -> SendTrueVehicleState/2(CommBusLocal), SendTargetStatus/2(CommBusLocal), VehicleStateSaveData/2(CommBusLocal), SendTrackList/2(CommBusLocal)
  SimmBusLocal/1 -> SendWeaponsRelease/2(SimmBusLocal), SendVehicleIsDead/2(SimmBusLocal), VehicleStateSaveData/3(SimmBusLocal), SendTrueVehicleState/3(SimmBusLocal), SendNewAssignment/2(SimmBusLocal)

== system cooperative/SendMessage/SendMessage/SendMessageMatlab ==
  Message : Inport
  Enable : EnablePort
  SendMessageS : S-Function  FunctionName=SendMessageS  Parameters='g_CommunicationMemory',MessageType,ReuseMatrix  EnableBusSupport=off
  wires:
  Message/1 -> SendMessageS/1

== system cooperative/SendTruth /SendMessage/SendMessageMatlab ==
  Message : Inport
  Enable : EnablePort
  SendMessageS : S-Function  FunctionName=SendMessageS  Parameters='g_TruthMemory',MessageType,ReuseMatrix  EnableBusSupport=off
  wires:
  Message/1 -> SendMessageS/1

== system cooperative/Target 1/AVDS Data/SaveTarget  Data for AVDS ==
  note: SaveTargetData for AVDS
      |
      | PURPOSE: Saves target state information to a text file that is suitable
      |      for playback in AVDS.
      | IMPLEMENTATION:
      | - AVDSData2WorkSpace - calls the M-function "AVDSData2WorkSpace"
      |      to save the data.
  Time : Inport  SampleTime=g_SampleTime
  ID : Inport  Port=2  SampleTime=g_SampleTime
  Data : Inport  Port=3  SampleTime=g_SampleTime
  Vehicle Type : Inport  Port=4  SampleTime=g_SampleTime
  Enable : EnablePort
  AVDSData2WorkSpaceS : S-Function  FunctionName=AVDSData2WorkSpaceS  EnableBusSupport=off
  Mux1 : Mux
  wires:
  Mux1/1 -> AVDSData2WorkSpaceS/1
  Time/1 -> Mux1/2
  ID/1 -> Mux1/1
  Data/1 -> Mux1/3
  Vehicle Type/1 -> Mux1/4

== system cooperative/Target 1/SendTargetState/Enabled Subsystem ==
  TargetState : Inport
  Enable : EnablePort
  Digital Clock : DigitalClock  SampleTime=g_SampleTime
  SaveTargetState : DataStoreWrite  DataStoreName=TargetState  SampleTime=g_SampleTime
  TimeStamp : Outport
  wires:
  Digital Clock/1 -> TimeStamp/1
  TargetState/1 -> SaveTargetState/1

== system cooperative/Target 1/SendTrueVehicleKilled/Enabled Subsystem ==
  VehicleKilled : Inport
  Enable : EnablePort
  Digital Clock : DigitalClock  SampleTime=g_SampleTime
  SaveVehicleKilled : DataStoreWrite  DataStoreName=VehicleKilled  SampleTime=g_SampleTime
  TimeStamp : Outport
  wires:
  VehicleKilled/1 -> SaveVehicleKilled/1
  Digital Clock/1 -> TimeStamp/1

== system cooperative/UAV1/EmbeddedFlightSoftware/CooperationManager ==
  note: Cooperation Manager
      |
      | PURPOSE: This manager is used to facilitate cooperation
      |      between the vehicles. At this time the only function
      |      implemented is the Assginment manager which calculates
      |      vehicle /task assignments.
      |
      | IMPLEMENTATION:
      | - Coordination Timing - adds a time delay before the assignment
      |      calculation to give other vehicles time to generate new plans.
      | - Calculate Assignment - this subsystem contains blocks used to
      |      calculate the vehicle/task assignments. This block is enabled
      |      by the signal "New Plans", after the Coordination Timing delay.
  SimBusIn : Inport  SampleTime=g_SampleTime
  ComBusIn : Inport  Port=2  SampleTime=g_SampleTime
  ComBusLocalIn : Inport  Port=3  SampleTime=g_SampleTime
  Enable : Inport  Port=4  SampleTime=g_SampleTime
  Bus Creator : BusCreator  Inputs=3
  Bus Creator1 : BusCreator  Inputs=1
  Calculate Assignment : Subsystem  TreatAsAtomicUnit=on
  Enable Reassignment : Subsystem
  Task List : Subsystem
  Terminator : Terminator
  ComBusOut : Outport
  SimBusOut : Outport  Port=2
  wires:
  Calculate Assignment/3(AuctionData) -> Bus Creator/3
  Calculate Assignment/2(Algorithm Data) -> Bus Creator/2
  Task List/1(UnassignTaskFlag) -> Terminator/1
  SimBusIn/1 -> Calculate Assignment/3(SimBusIn)
  Enable Reassignment/1(Enable Reassignment) -> Calculate Assignment/Enable
  Enable/1 -> Enable Reassignment/1(Enable)
  ComBusLocalIn/1 -> Task List/1(ComBusLocalIn), Enable Reassignment/2(ComBusLocalIn), Calculate Assignment/1(ComBusLocalIn)  "Local Bus"
  ComBusIn/1 -> Enable Reassignment/3(ComBusIn), Calculate Assignment/2(ComBusIn)
  Calculate Assignment/1(Local Assignment) -> Bus Creator/1  "Assignment"
  Bus Creator/1 -> ComBusOut/1  "CooperationManager(com)"
  Calculate Assignment/4(NewAssignmetTime) -> Bus Creator1/1  "NewAssignmentTime"
  Bus Creator1/1 -> SimBusOut/1  "CooperationManager(com)"

== system cooperative/UAV1/EmbeddedFlightSoftware/RouteManager ==
  note: Route Manager
      |
      | PURPOSE: This manager is used to plan and select the route for the
      |      vehicle to fly.
      |
      | Implementation:
      | - Replan - when enabled, calculates the lowest cost route to all known targets,
      |      based on each target's state. Replan is enabled If any of the vehicles report
      |      "Task Finished" or if any of the targets change state,
      | - RouteSelection - calls the function "RouteSelection" to implement waypoints
      |      for the route selected for this vehicle during the vehicle/target assignment in
      |      the cooperation manager.
      | - Task Status - monitors the status of the vehicle's assigned task.
  SimBusIn : Inport  SampleTime=g_SampleTime
  ComBusIn : Inport  Port=2  SampleTime=g_SampleTime
  SimBusLocalIn : Inport  Port=3  SampleTime=g_SampleTime
  ComBusLocalIn : Inport  Port=4  SampleTime=g_SampleTime
  Enable : Inport  Port=5  SampleTime=g_SampleTime
  Bus Creator : BusCreator  Inputs=1
  Bus Creator1 : BusCreator  Inputs=3
  Constant : Constant  Value=g_AssignmentAlgorithm
  Constant1 : Constant  Value=g_TypeAssignment.CapTransShip
  Logical Operator : Logic
  Relational Operator : RelationalOperator  Operator===  InputSameDT=on
  ReplanSingle : Subsystem
  Task Status : Subsystem
  SimBusOut : Outport
  ComBusOut : Outport  Port=2
  wires:
  Constant1/1 -> Relational Operator/2
  Constant/1 -> Relational Operator/1
  Relational Operator/1 -> Logical Operator/1
  Logical Operator/1 -> ReplanSingle/3(Enable)
  Enable/1 -> Task Status/2(Enable), Logical Operator/2
  ReplanSingle/1(NewPlans) -> Bus Creator1/1
  Bus Creator/1 -> SimBusOut/1  "RouteManager(sim)"
  ComBusIn/1 -> ReplanSingle/1(ComBusIn)
  Task Status/1(Task Status) -> Bus Creator1/3
  Task Status/2(Vehicle Finished) -> Bus Creator/1
  SimBusIn/1 -> ReplanSingle/4(SimBusIn), Task Status/3(SimBusIn)
  ReplanSingle/2(ReplanETAsCosts) -> Bus Creator1/2
  Bus Creator1/1 -> ComBusOut/1  "RouteManager(com)"
  ComBusLocalIn/1 -> Task Status/1(Local (Comm)), ReplanSingle/2(ComBusLocalIn)  "Local Bus"
  SimBusLocalIn/1 -> ReplanSingle/5(SimBusLocalIn)  "Vehicle (Sim)"

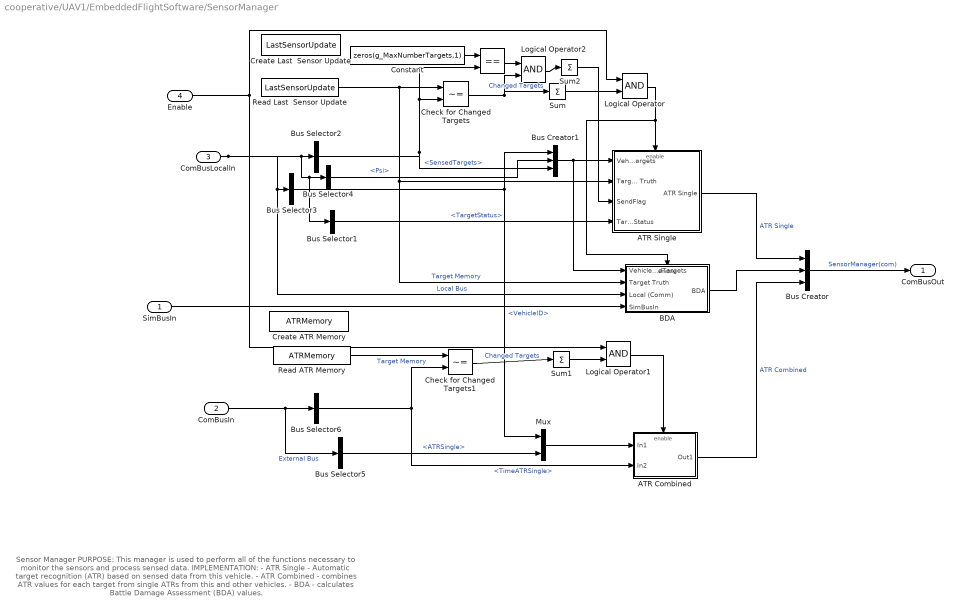
== system cooperative/UAV1/EmbeddedFlightSoftware/SensorManager ==
  note: Sensor Manager
      |
      | PURPOSE: This manager is used to perform all of the functions
      | necessary to monitor the sensors and process sensed data.
      |
      | IMPLEMENTATION:
      | - ATR Single - Automatic target recognition (ATR) based on sensed data
      |      from this vehicle.
      | - ATR Combined - combines ATR values for each target from single ATRs
      |      from this and other vehicles.
      | - BDA - calculates Battle Damage Assessment (BDA) values.
  SimBusIn : Inport  SampleTime=g_SampleTime
  ComBusIn : Inport  Port=2  SampleTime=g_SampleTime
  ComBusLocalIn : Inport  Port=3  SampleTime=g_SampleTime
  Enable : Inport  Port=4  SampleTime=g_SampleTime
  " " : RelationalOperator  Operator===  InputSameDT=on
  ATR Combined : Subsystem  TreatAsAtomicUnit=on
  ATR Single : Subsystem  TreatAsAtomicUnit=on
  BDA : Subsystem  TreatAsAtomicUnit=on
  Bus Creator : BusCreator  Inputs=3
  Bus Creator1 : BusCreator  Inputs=3
  Bus Selector1 : BusSelector  OutputSignals=EFS(com).TargetManager(com).Target Status.TargetStatus
  Bus Selector2 : BusSelector  OutputSignals=Dynamics(com).SensedTargets.SensedTargets
  Bus Selector3 : BusSelector  OutputSignals=VehicleID
  Bus Selector4 : BusSelector  OutputSignals=Dynamics(com).AC Dynamics.Psi
  Bus Selector5 : BusSelector  OutputSignals=ATRSingle
  Bus Selector6 : BusSelector  OutputSignals=TimeATRSingle
  Check for Changed Targets : RelationalOperator  Operator=~=  InputSameDT=on
  Check for Changed Targets1 : RelationalOperator  Operator=~=  InputSameDT=on
  Constant : Constant  Value=zeros(g_MaxNumberTargets,1)
  Create ATR Memory : DataStoreMemory  DataStoreName=ATRMemory  InitialValue=1
  Create Last  Sensor Update : DataStoreMemory  DataStoreName=LastSensorUpdate  InitialValue=zeros(g_MaxNumberTargets,1)
  Logical Operator : Logic
  Logical Operator1 : Logic
  Logical Operator2 : Logic
  Mux : Mux  Inputs=2
  Read ATR Memory : DataStoreRead  DataStoreName=ATRMemory  SampleTime=g_SampleTime
  Read Last  Sensor Update : DataStoreRead  DataStoreName=LastSensorUpdate  SampleTime=g_SampleTime
  Sum : Sum  Inputs=|+  SaturateOnIntegerOverflow=on  InputSameDT=on  OutDataTypeStr=Inherit: Same as first input
  Sum1 : Sum  Inputs=|+  SaturateOnIntegerOverflow=on  InputSameDT=on  OutDataTypeStr=Inherit: Same as first input
  Sum2 : Sum  Inputs=|+  SaturateOnIntegerOverflow=on  InputSameDT=on  OutDataTypeStr=Inherit: Same as first input
  ComBusOut : Outport
  wires:
  Bus Selector1/1 -> ATR Single/4(TargetStatus)  "<TargetStatus>"
  Sum2/1 -> ATR Single/3(SendFlag)
  Logical Operator2/1 -> Sum2/1
  " "/1 -> Logical Operator2/1
  Constant/1 -> " "/1
  Enable/1 -> Logical Operator1/1, Logical Operator/1
  Logical Operator1/1 -> ATR Combined/Enable
  Sum1/1 -> Logical Operator1/2
  Logical Operator/1 -> BDA/Enable, ATR Single/Enable
  Sum/1 -> Logical Operator/2
  ATR Single/1(ATR Single) -> Bus Creator/1  "ATR Single"
  BDA/1(BDA) -> Bus Creator/2
  Bus Creator/1 -> ComBusOut/1  "SensorManager(com)"
  ATR Combined/1(Out1) -> Bus Creator/3  "ATR Combined"
  Bus Selector6/1 -> ATR Combined/2(In2), Check for Changed Targets1/2  "<TimeATRSingle>"
  Mux/1 -> ATR Combined/1(In1)
  Bus Selector5/1 -> Mux/2  "<ATRSingle>"
  ComBusIn/1 -> Bus Selector5/1, Bus Selector6/1  "External Bus"
  Bus Selector4/1 -> Bus Creator1/2  "<Psi>"
  Bus Selector3/1 -> Mux/1, Bus Creator1/1  "<VehicleID>"
  Bus Selector2/1 -> " "/2, Check for Changed Targets/2, Bus Creator1/3  "<SensedTargets>"
  Bus Creator1/1 -> BDA/1(VehicleID Psi SensedTargets), ATR Single/1(VehicleID Psi SensedTargets)
  ComBusLocalIn/1 -> BDA/3(Local (Comm)), Bus Selector3/1, Bus Selector1/1, Bus Selector4/1, Bus Selector2/1  "Local Bus"
  Read ATR Memory/1 -> Check for Changed Targets1/1  "Target Memory"
  Check for Changed Targets1/1 -> Sum1/1  "Changed Targets"
  Read Last  Sensor Update/1 -> BDA/2(Target Truth), ATR Single/2(Target Truth), Check for Changed Targets/1  "Target Memory"
  Check for Changed Targets/1 -> Logical Operator2/2, Sum/1  "Changed Targets"
  SimBusIn/1 -> BDA/4(SimBusIn)

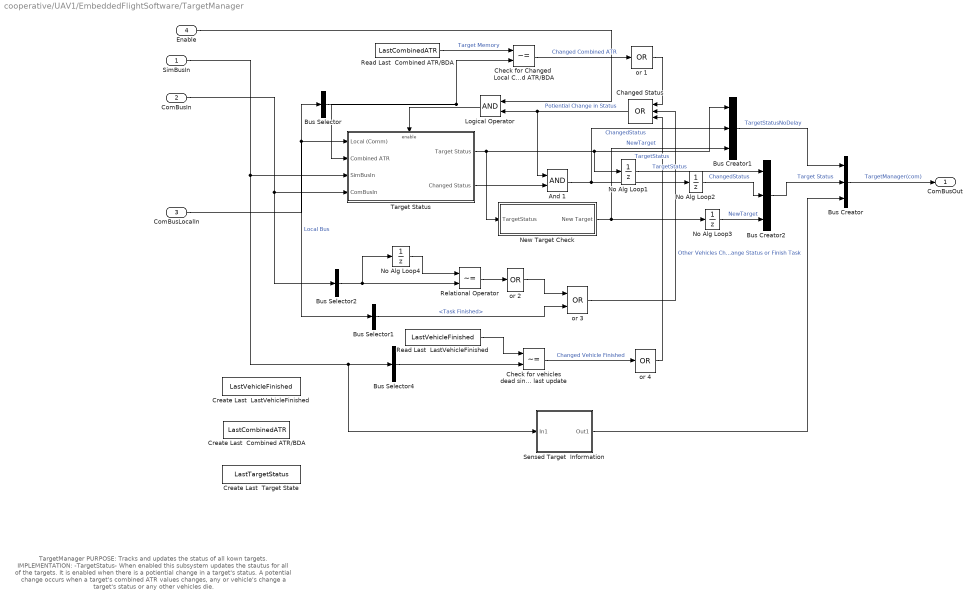
== system cooperative/UAV1/EmbeddedFlightSoftware/TargetManager ==
  note: TargetManager
      |
      | PURPOSE: Tracks and updates the status of all
      |      kown targets.
      |
      | IMPLEMENTATION:
      | -TargetStatus- When enabled this subsystem updates the stautus for all of the targets.
      |      It is enabled when there is a potiential change in a target's status. A potential
      |      change occurs when a target's combined ATR values changes, any or vehicle's
      |      change a target's status or any other vehicles die.
  SimBusIn : Inport  SampleTime=g_SampleTime
  ComBusIn : Inport  Port=2  SampleTime=g_SampleTime
  ComBusLocalIn : Inport  Port=3  SampleTime=g_SampleTime
  Enable : Inport  Port=4  SampleTime=g_SampleTime
  And 1 : Logic
  Bus Creator : BusCreator  Inputs=3
  Bus Creator1 : BusCreator  Inputs=3
  Bus Creator2 : BusCreator  Inputs=3
  Bus Selector : BusSelector  OutputSignals=EFS(com).SensorManager(com).ATR Combined.CombinedATRValues,EFS(com).SensorManager(com).BDA  OutputAsBus=on
  Bus Selector1 : BusSelector  OutputSignals=EFS(com).RouteManager(com).TaskStatus.Task Finished
  Bus Selector2 : BusSelector  OutputSignals=TimeChangedStatus,TimeTargetAttacked  OutputAsBus=on
  Bus Selector4 : BusSelector  OutputSignals=ExternalTruth.VehicleIsDead  OutputAsBus=on
  Changed Status : Logic  Operator=OR  Inputs=3
  Check for Changed  Local Combined ATR/BDA : RelationalOperator  Operator=~=  InputSameDT=on
  Check for vehicles dead since last update : RelationalOperator  Operator=~=  InputSameDT=on
  Create Last  Combined ATR/BDA : DataStoreMemory  DataStoreName=LastCombinedATR  InitialValue=[1:(g_MaxNumberTargets*2)]*0
  Create Last  LastVehicleFinished : DataStoreMemory  DataStoreName=LastVehicleFinished  InitialValue=[1:(g_MaxNumberVehicles)]*0
  Create Last  Target State : DataStoreMemory  DataStoreName=LastTargetStatus  InitialValue=[1:(g_MaxNumberTargets)]*0
  Logical Operator : Logic
  New Target Check : Subsystem
  No Alg Loop{1..4} (4 alike) : UnitDelay  SampleTime=g_SampleTime
  Read Last  Combined ATR/BDA : DataStoreRead  DataStoreName=LastCombinedATR  SampleTime=g_SampleTime
  Read Last  LastVehicleFinished : DataStoreRead  DataStoreName=LastVehicleFinished  SampleTime=g_SampleTime
  Relational Operator : RelationalOperator  Operator=~=  InputSameDT=on
  Sensed Target  Information : Subsystem
  Target Status : Subsystem  TreatAsAtomicUnit=on
  or 1 : Logic  Operator=OR  Inputs=1
  or 2 : Logic  Operator=OR  Inputs=1
  or 3 : Logic  Operator=OR
  or 4 : Logic  Operator=OR  Inputs=1
  ComBusOut : Outport
  wires:
  or 2/1 -> or 3/1
  No Alg Loop4/1 -> Relational Operator/1
  No Alg Loop3/1 -> Bus Creator2/3  "NewTarget"
  No Alg Loop2/1 -> Bus Creator2/2  "ChangedStatus"
  No Alg Loop1/1 -> Bus Creator2/1  "TargetStatus"
  New Target Check/1(New Target) -> No Alg Loop3/1, Bus Creator1/3  "NewTarget"
  Sensed Target  Information/1(Out1) -> Bus Creator/3
  Enable/1 -> Logical Operator/1
  Logical Operator/1 -> Target Status/Enable
  Bus Selector4/1 -> Check for vehicles dead since last update/2
  Read Last  LastVehicleFinished/1 -> Check for vehicles dead since last update/1
  Check for vehicles dead since last update/1 -> or 4/1  "Changed Vehicle Finished"
  or 4/1 -> Changed Status/3
  or 3/1 -> Changed Status/2  "Other Vehicles Change Status or Finish Task"
  Relational Operator/1 -> or 2/1
  Bus Selector1/1 -> or 3/2  "<Task Finished>"
  Check for Changed  Local Combined ATR/BDA/1 -> or 1/1  "Changed Combined ATR"
  Target Status/1(Target Status) -> No Alg Loop1/1, Bus Creator1/1, New Target Check/1(TargetStatus)  "TargetStatus"
  Bus Creator2/1 -> Bus Creator/2  "Target Status"
  Changed Status/1 -> Logical Operator/2, And 1/1  "Potiential Change in Status"
  Bus Selector2/1 -> Relational Operator/2, No Alg Loop4/1
  or 1/1 -> Changed Status/1
  Bus Selector/1 -> Target Status/2(Combined ATR), Check for Changed  Local Combined ATR/BDA/2
  Read Last  Combined ATR/BDA/1 -> Check for Changed  Local Combined ATR/BDA/1  "Target Memory"
  Target Status/2(Changed Status) -> And 1/2
  And 1/1 -> Bus Creator1/2, No Alg Loop2/1  "ChangedStatus"
  ComBusIn/1 -> Bus Selector2/1, Target Status/4(ComBusIn)
  Bus Creator/1 -> ComBusOut/1  "TargetManager(com)"
  SimBusIn/1 -> Sensed Target  Information/1(In1), Bus Selector4/1, Target Status/3(SimBusIn)
  ComBusLocalIn/1 -> Bus Selector1/1, Bus Selector/1, Target Status/1(Local (Comm))  "Local Bus"
  Bus Creator1/1 -> Bus Creator/1  "TargetStatusNoDelay"

== system cooperative/UAV1/EmbeddedFlightSoftware/WeaponsManager ==
  note: Weapons Manager
      |
      | PURPOSE: Selects a weapon and then simulates its deployment.
      |
      | IMPLEMENTATION:
      | -TargetBombed- calls the function "WeaponsRelease.m" which returns
      |      a unique BombID number, the type of bomb dropped and the
      |      bomb's impact coordinates.
  ComBusLocalIn : Inport  SampleTime=g_SampleTime
  Enable : EnablePort
  Bus Creator : BusCreator  Inputs=1
  Bus Creator1 : BusCreator  Inputs=1
  Bus Creator2 : BusCreator
  Bus Selector : BusSelector  OutputSignals=VehicleID,EFS(com).RouteManager(com).TaskStatus.Target Attacked,Dynamics(com).AC Dynamics.Position_x,Dynamics(com).AC Dynamics.Position_y  OutputAsBus=on
  Constant : Constant  Value=0
  Demux : Demux
  TargetBombed : S-Function  FunctionName=WeaponsReleaseS  Parameters='Bomb'  EnableBusSupport=off
  SimBusOut : Outport
  ComBusOut : Outport  Port=2  InitialOutput=[0]
  wires:
  Bus Selector/1 -> TargetBombed/1
  Bus Creator2/1 -> Bus Creator1/1  "BombDrop"
  Bus Creator1/1 -> SimBusOut/1  "WeaponsManager(sim)"
  Demux/4 -> Bus Creator2/4  "BombPositionY"
  Demux/3 -> Bus Creator2/3  "BombPositionX"
  Demux/2 -> Bus Creator2/2  "BombType"
  Demux/1 -> Bus Creator2/1  "BombID"
  TargetBombed/1 -> Demux/1
  Constant/1 -> Bus Creator/1  "WeaponsManagerTemp"
  Bus Creator/1 -> ComBusOut/1  "WeaponsManager(com)"
  ComBusLocalIn/1 -> Bus Selector/1

== system cooperative/UAV1/ReceiveTruth/ImplementNewAssignment ==
  VehicleID : Inport
  TruthBus : Inport  Port=2
  Constant : Constant  Value=0
  Relational Operator : RelationalOperator  Operator=<  InputSameDT=on
  VehicleAlive : Subsystem  TreatAsAtomicUnit=on
  wires:
  TruthBus/1 -> VehicleAlive/2(In2)
  Constant/1 -> Relational Operator/1
  VehicleID/1 -> VehicleAlive/1(In1), Relational Operator/2
  Relational Operator/1 -> VehicleAlive/Enable

== system cooperative/UAV1/SaveAVDSData/SaveVehicleData for AVDS ==
  note: SaveVehicleData for AVDS
      |
      | PURPOSE: Saves vehicle state information to a text file that is suitable
      |      for playback in AVDS.
      | IMPLEMENTATION:
      | - AVDSData2WorkSpace - calls the M-function "AVDSData2WorkSpace"
      |      to save the data.
  Time : Inport  SampleTime=g_SampleTime
  ID : Inport  Port=2  SampleTime=g_SampleTime
  Data : Inport  Port=3  SampleTime=g_SampleTime
  Vehicle Type : Inport  Port=4  SampleTime=g_SampleTime
  Enable : EnablePort
  AVDSData2WorkSpaceS : S-Function  FunctionName=AVDSData2WorkSpaceS  EnableBusSupport=off
  Mux1 : Mux
  wires:
  Vehicle Type/1 -> Mux1/4
  Data/1 -> Mux1/3
  ID/1 -> Mux1/1
  Time/1 -> Mux1/2
  Mux1/1 -> AVDSData2WorkSpaceS/1

== system cooperative/UAV1/SendMessages/SendATRSingle ==
  VehicleID : Inport
  CommBusLocal : Inport  Port=2
  Bus Selector4 : BusSelector  OutputSignals=EFS(com).SensorManager(com).ATR Single.ATR Time,EFS(com).SensorManager(com).ATR Single  OutputAsBus=on
  Mux3 : Mux  Inputs=3
  SendATRSingle : cooperative/SendMessage  ReuseMatrix=growing  MessageTypeStr=ATRSingle
  Terminator : Terminator
  VehicleOffset : Constant  Value=g_ObjectMessageIDs.AllVehiclesTypeShifted + 1
  wires:
  CommBusLocal/1 -> Bus Selector4/1
  VehicleID/1 -> Mux3/1
  Mux3/1 -> SendATRSingle/1
  Bus Selector4/1 -> Mux3/2
  VehicleOffset/1 -> Mux3/3
  SendATRSingle/1 -> Terminator/1
